simulink model "Pendel"  (R2017b)
settings: Solver=VariableStepAuto  StartTime=0.0  StopTime=100  RelTol=1e-3
libraries: vrlib x2
settings Model: Creator=aby032  LastModifiedBy=aby032

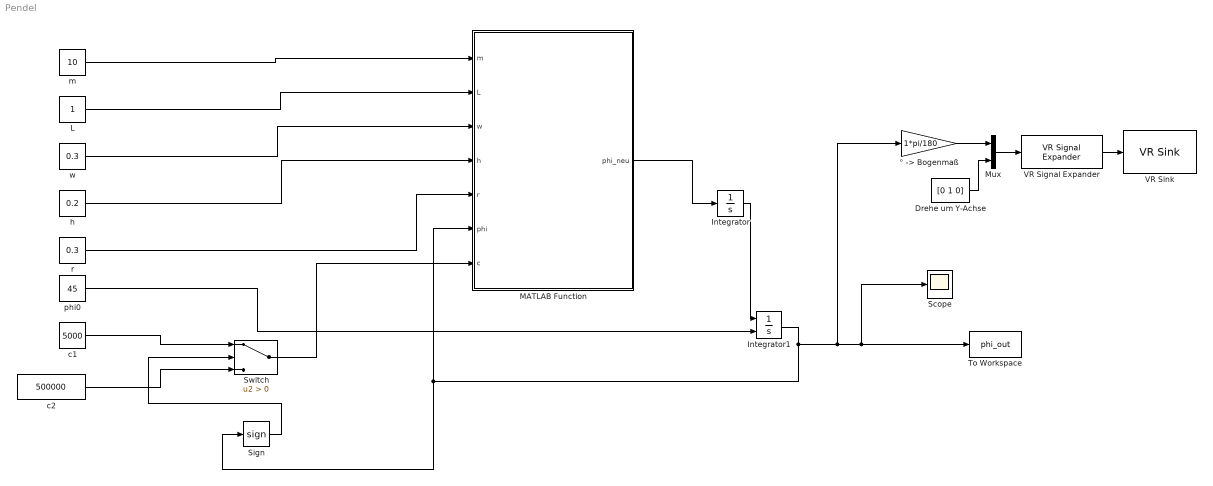
== system Pendel ==
  Drehe um Y-Achse : Constant  Value=[0 1 0]
  Integrator : Integrator
  Integrator1 : Integrator  InitialConditionSource=external
  L : Constant
  MATLAB Function : MATLAB Function  TreatAsAtomicUnit=on
  Mux : Mux  Inputs=2
  Scope : Scope
  Sign : Signum
  Switch : Switch  Criteria=u2 > Threshold
  To Workspace : ToWorkspace  VariableName=phi_out  SaveFormat=Timeseries  SampleTime=-1
  VR Signal Expander : vrlib/VR Signal Expander  outwidth=4  outidx=[4 1 2 3]
      settings: SourceProductName=Simulink 3D Animation  SourceProductBaseCode=VR
  VR Sink : vrlib/VR Sink  InstantiateOnLoad=on  SampleTime=0.005  ViewEnable=on  RemoteChange=off  RemoteView=on  FieldsWritten=Seiltrommel.rotation.4.1.1.double  WorldFileName=CrazyPendlm.wrl  AutoView=off  VideoDimensions=[]  AllowVariableSize=off
      settings: SourceProductBaseCode=VR
  c1 : Constant  Value=5000
  c2 : Constant  Value=500000
  h : Constant  Value=0.2
  m : Constant  Value=10
  phi0 : Constant  Value=45
  r : Constant  Value=0.3
  w : Constant  Value=0.3
  "° -> Bogenmaß" : Gain  Gain=1*pi/180
  wires:
  Integrator1/1 -> "° -> Bogenmaß"/1, Scope/1, To Workspace/1, Sign/1, MATLAB Function/6(phi)
  Sign/1 -> Switch/2
  c2/1 -> Switch/3
  c1/1 -> Switch/1
  m/1 -> MATLAB Function/1(m)
  L/1 -> MATLAB Function/2(L)
  w/1 -> MATLAB Function/3(w)
  h/1 -> MATLAB Function/4(h)
  r/1 -> MATLAB Function/5(r)
  MATLAB Function/1(phi_neu) -> Integrator/1
  Integrator/1 -> Integrator1/1
  phi0/1 -> Integrator1/2
  Switch/1 -> MATLAB Function/7(c)
  VR Signal Expander/1 -> VR Sink/1
  Drehe um Y-Achse/1 -> Mux/2
  Mux/1 -> VR Signal Expander/1
  "° -> Bogenmaß"/1 -> Mux/1

== matlab function Pendel/MATLAB Function ==
  data: m input; phi_neu output; L input; w input; h input; r input; phi input; c input
function phi_neu = fcn(m,L,w,h,r,phi,c)
g = 9.80665;                    %Erdbeschleunigung

Fp = m*g*sind(phi);             %Kraft Pendel
s = (L+h/2);                    %Abstand Drehachse - Quader
Mp = Fp*s;                      %Drehmoment Pendel duch Quader verursacht


cs = deg2rad(phi)*r;            %Abstand um den Feder gezogen wird Betrag
Ff = c*cs;                      %Federkraft
Ms = Ff*r;                      %Drehmoment Pendel duch Feder


Mg = Mp - Ms;                   %Gesamtdrehmoment

Jp = 1/12 * m *(h*h + w*w);     %Massenträgheitsmoment Quader
Jg = Jp+m*s*s                   %Massenträgheitsmoment in Bezug zu Drehachse

phi_neu = rad2deg(Mg/Jg);
